simulink model "SAME5x_EXpicGUI_base"  (R2020b)
(part 2 of 3)

      mask TypeOptions FPLLMULT: PLL Multiply by 128 | PLL Multiply by 127 | PLL Multiply by 126 | PLL Multiply by 125 | PLL Multiply by 124 | PLL Multiply by 123 | PLL Multiply by 122 | PLL Multiply by 121 | PLL Multiply by 120 | PLL Multiply by 119 | PLL Multiply by 118 | PLL Multiply by 117 | PLL Multiply by 116 | PLL Multiply by 115 | PLL Multiply by 114 | PLL Multiply by 113 | PLL Multiply by 112 | PLL Multiply by 111 | PLL Multiply by 110 | PLL Multiply by 109 | PLL Multiply by 108 | PLL Multiply by 107 | PLL Multiply by 106 | PLL Multiply by 105 | PLL Multiply by 104 | PLL Multiply by 103 | PLL Multiply by 102 | PLL Multiply by 101 | PLL Multiply by 100 | PLL Multiply by 99 | PLL Multiply by 98 | PLL Multiply by 97 | PLL Multiply by 96 | PLL Multiply by 95 | PLL Multiply by 94 | PLL Multiply by 93 | PLL Multiply by 92 | PLL Multiply by 91 | PLL Multiply by 90 | PLL Multiply by 89 | PLL Multiply by 88 | PLL Multiply by 87 | PLL Multiply by 86 | PLL Multiply by 85 | PLL Multiply by 84 | PLL Multiply by 83 | PLL Multiply by 82 | PLL Multiply by 81 | PLL Multiply by 80 | PLL Multiply by 79 | PLL Multiply by 78 | PLL Multiply by 77 | PLL Multiply by 76 | PLL Multiply by 75 | PLL Multiply by 74 | PLL Multiply by 73 | PLL Multiply by 72 | PLL Multiply by 71 | PLL Multiply by 70 | PLL Multiply by 69 | PLL Multiply by 68 | PLL Multiply by 67 | PLL Multiply by 66 | PLL Multiply by 65 | PLL Multiply by 64 | PLL Multiply by 63 | PLL Multiply by 62 | PLL Multiply by 61 | PLL Multiply by 60 | PLL Multiply by 59 | PLL Multiply by 58 | PLL Multiply by 57 | PLL Multiply by 56 | PLL Multiply by 55 | PLL Multiply by 54 | PLL Multiply by 53 | PLL Multiply by 52 | PLL Multiply by 51 | PLL Multiply by 50 | PLL Multiply by 49 | PLL Multiply by 48 | PLL Multiply by 47 | PLL Multiply by 46 | PLL Multiply by 45 | PLL Multiply by 44 | PLL Multiply by 43 | PLL Multiply by 42 | PLL Multiply by 41 | PLL Multiply by 40 | PLL Multiply by 39 | PLL Multiply by 38 | PLL Multiply by 37 | PLL Multiply by 36 | PLL Multiply by 35 | PLL Multiply by 34 | PLL Multiply by 33 | PLL Multiply by 32 | PLL Multiply by 31 | PLL Multiply by 30 | PLL Multiply by 29 | PLL Multiply by 28 | PLL Multiply by 27 | PLL Multiply by 26 | PLL Multiply by 25 | PLL Multiply by 24 | PLL Multiply by 23 | PLL Multiply by 22 | PLL Multiply by 21 | PLL Multiply by 20 | PLL Multiply by 19 | PLL Multiply by 18 | PLL Multiply by 17 | PLL Multiply by 16 | PLL Multiply by 15 | PLL Multiply by 14 | PLL Multiply by 13 | PLL Multiply by 12 | PLL Multiply by 11 | PLL Multiply by 10 | PLL Multiply by 9 | PLL Multiply by 8 | PLL Multiply by 7 | PLL Multiply by 6 | PLL Multiply by 5 | PLL Multiply by 4 | PLL Multiply by 3 | PLL Multiply by 2 | PLL Multiply by 1
      mask TypeOptions UPLLFSEL: USB PLL input is 24 MHz | USB PLL input is 12 MHz
      mask TypeOptions DMTINTV: Window/Interval value is 127/128 counter value | Window/Interval value is 63/64 counter value | Window/Interval value is 31/32 counter value | Window/Interval value is 15/16 counter value | Window/Interval value is 7/8 counter value | Window/Interval value is 3/4 counter value | Window/Interval value is 1/2 counter value | Window/Interval value is zero
      mask TypeOptions WDTSPGM: WDT stops during Flash programming | WDT runs during Flash programming
      mask TypeOptions FDMTEN: Deadman Timer is enabled | Deadman Timer is disabled
      mask TypeOptions TRCEN: Trace features in the CPU are enabled | Trace features in the CPU are disabled
      mask TypeOptions BOOTISA: Boot code and Exception code is MIPS32 | Boot code and Exception code is microMIPS
      mask TypeOptions FECCCON: ECC and Dynamic ECC are disabled (ECCCON<1:0> bits are writable) | ECC and Dynamic ECC are disabled (ECCCON<1:0> bits are locked) | Dynamic Flash ECC is enabled (ECCCON<1:0> bits are locked) | Flash ECC is enabled (ECCCON<1:0> bits are locked; disables word Flash writes) | ECC and Dynamic ECC are disabled (ECCCON bits are writable) | ECC and Dynamic ECC are disabled (ECCCON bits are locked) | Dynamic Flash ECC is enabled (ECCCON bits are locked) | Flash ECC is enabled (ECCCON bits are locked)
      mask TypeOptions EXTDDRSIZE: Not used
      mask TypeOptions FSLEEP: Flash is powered down when the device is in Sleep mode | Flash power down is controlled by the VREGS bit
      mask TypeOptions DBGPER: Allow CPU access to all permission regions | PG0: Deny PG1: Allow PG2: Allow | PG0: Allow PG1: Deny PG2: Allow | Allow CPU access to Permission Group 2 permission regions | PG0: Allow PG1: Allow PG2: Deny | Allow CPU access to Permission Group 1 permission regions | Allow CPU access to Permission Group 0 permission regions | Deny CPU access to all permission regions
      mask TypeOptions EJTAGBEN: Normal EJTAG functionality | Reduced EJTAG functionality
      mask TypeOptions TSEQ: Not used
      mask TypeOptions CSEQ: Not used
      mask TypeOptions RWDTPS: 1:1048576 | 1:524288 | 1:262144 | 1:131072 | 1:65536 | 1:32768 | 1:16384 | 1:8192 | 1:4096 | 1:2048 | 1:1024 | 1:512 | 1:256 | 1:128 | 1:64 | 1:32 | 1:16 | 1:8 | 1:4 | 1:2 | 1:1 | 1:2147483648 | 1:1073741824 | 1:536870912 | 1:268435456 | 1:134217728 | 1:67108864 | 1:33554432 | 1:16777216 | 1:8388608 | 1:4194304 | 1:2097152
      mask TypeOptions RCLKSEL: Always use LPRC | Use FRC when WINDIS = 0; system clock is not INTOSC/LPRC and device is not in Sleep;otherwise; use INTOSC/LPRC | Use peripheral clk when system clock is not INTOSC/LPRC and device is not in Sleep;otherwise; use INTOSC/LPRC | Always use BFRC/256 | Use FRC when WINDIS = 0 and device is not in Sleep; otherwise; use BFRC/256 | Use peripheral clk when device is not in Sleep; otherwise; use BFRC/256
      mask TypeOptions SWDTPS: 1:1048576 | 1:524288 | 1:262144 | 1:131072 | 1:65536 | 1:32768 | 1:16384 | 1:8192 | 1:4096 | 1:2048 | 1:1024 | 1:512 | 1:256 | 1:128 | 1:64 | 1:32 | 1:16 | 1:8 | 1:4 | 1:2 | 1:1 | 1:2147483648 | 1:1073741824 | 1:536870912 | 1:268435456 | 1:134217728 | 1:67108864 | 1:33554432 | 1:16777216 | 1:8388608 | 1:4194304 | 1:2097152
      mask TypeOptions DMTIVTL: Not used
      mask TypeOptions DMTIVTH: Not used
      mask TypeOptions DMTCNTL: Not used
      mask TypeOptions DMTCNTH: Not used
      mask TypeOptions DMTDIS: Dead Man Timer is Disabled and can be enabled by software | Dead Man Timer is Enabled and cannot be disabled by software
      mask TypeOptions SMBEN: SMBus input threshold is enabled | Standard I2C input threshold operation
      mask TypeOptions SPI2PIN: SPI2 uses I/O remap (PPS) pins | SPI2 uses dedicated I/O pins
      mask TypeOptions CTXT3: Not Assigned | Alternate Register set assigned to IPL level 7 | Alternate Register set assigned to IPL level 6 | Alternate Register set assigned to IPL level 5 | Alternate Register set assigned to IPL level 4 | Alternate Register set assigned to IPL level 3 | Alternate Register set assigned to IPL level 2 | Alternate Register set assigned to IPL level 1
      mask TypeOptions CTXT4: Not Assigned | Alternate Register set assigned to IPL level 7 | Alternate Register set assigned to IPL level 6 | Alternate Register set assigned to IPL level 5 | Alternate Register set assigned to IPL level 4 | Alternate Register set assigned to IPL level 3 | Alternate Register set assigned to IPL level 2 | Alternate Register set assigned to IPL level 1
      mask TypeOptions MBXM0: Mailbox register configured for Master data read (Slave to Master data transfer) | Mailbox register configured for Master data write (Master to Slave data transfer)
      mask TypeOptions MBXM1: Mailbox register configured for Master data read (Slave to Master data transfer) | Mailbox register configured for Master data write (Master to Slave data transfer)
      mask TypeOptions MBXM2: Mailbox register configured for Master data read (Slave to Master data transfer) | Mailbox register configured for Master data write (Master to Slave data transfer)
      mask TypeOptions MBXM3: Mailbox register configured for Master data read (Slave to Master data transfer) | Mailbox register configured for Master data write (Master to Slave data transfer)
      mask TypeOptions MBXM4: Mailbox register configured for Master data read (Slave to Master data transfer) | Mailbox register configured for Master data write (Master to Slave data transfer)
      mask TypeOptions MBXM5: Mailbox register configured for Master data read (Slave to Master data transfer) | Mailbox register configured for Master data write (Master to Slave data transfer)
      mask TypeOptions MBXM6: Mailbox register configured for Master data read (Slave to Master data transfer) | Mailbox register configured for Master data write (Master to Slave data transfer)
      mask TypeOptions MBXM7: Mailbox register configured for Master data read (Slave to Master data transfer) | Mailbox register configured for Master data write (Master to Slave data transfer)
      mask TypeOptions MBXM8: Mailbox register configured for Master data read (Slave to Master data transfer) | Mailbox register configured for Master data write (Master to Slave data transfer)
      mask TypeOptions MBXM9: Mailbox register configured for Master data read (Slave to Master data transfer) | Mailbox register configured for Master data write (Master to Slave data transfer)
      mask TypeOptions MBXM10: Mailbox register configured for Master data read (Slave to Master data transfer) | Mailbox register configured for Master data write (Master to Slave data transfer)
      mask TypeOptions MBXM11: Mailbox register configured for Master data read (Slave to Master data transfer) | Mailbox register configured for Master data write (Master to Slave data transfer)
      mask TypeOptions MBXM12: Mailbox register configured for Master data read (Slave to Master data transfer) | Mailbox register configured for Master data write (Master to Slave data transfer)
      mask TypeOptions MBXM13: Mailbox register configured for Master data read (Slave to Master data transfer) | Mailbox register configured for Master data write (Master to Slave data transfer)
      mask TypeOptions MBXM14: Mailbox register configured for Master data read (Slave to Master data transfer) | Mailbox register configured for Master data write (Master to Slave data transfer)
      mask TypeOptions MBXM15: Mailbox register configured for Master data read (Slave to Master data transfer) | Mailbox register configured for Master data write (Master to Slave data transfer)
      mask TypeOptions MBXHSA: MSIxMBXD15 assigned to mailbox handshake protocol block A | MSIxMBXD14 assigned to mailbox handshake protocol block A | MSIxMBXD13 assigned to mailbox handshake protocol block A | MSIxMBXD12 assigned to mailbox handshake protocol block A | MSIxMBXD11 assigned to mailbox handshake protocol block A | MSIxMBXD10 assigned to mailbox handshake protocol block A | MSIxMBXD9 assigned to mailbox handshake protocol block A | MSIxMBXD8 assigned to mailbox handshake protocol block A | MSIxMBXD7 assigned to mailbox handshake protocol block A | MSIxMBXD6 assigned to mailbox handshake protocol block A | MSIxMBXD5 assigned to mailbox handshake protocol block A | MSIxMBXD4 assigned to mailbox handshake protocol block A | MSIxMBXD3 assigned to mailbox handshake protocol block A | MSIxMBXD2 assigned to mailbox handshake protocol block A | MSIxMBXD1 assigned to mailbox handshake protocol block A | MSIxMBXD0 assigned to mailbox handshake protocol block A
      mask TypeOptions MBXHSB: MSIxMBXD15 assigned to mailbox handshake protocol block B | MSIxMBXD14 assigned to mailbox handshake protocol block B | MSIxMBXD13 assigned to mailbox handshake protocol block B | MSIxMBXD12 assigned to mailbox handshake protocol block B | MSIxMBXD11 assigned to mailbox handshake protocol block B | MSIxMBXD10 assigned to mailbox handshake protocol block B | MSIxMBXD9 assigned to mailbox handshake protocol block B | MSIxMBXD8 assigned to mailbox handshake protocol block B | MSIxMBXD7 assigned to mailbox handshake protocol block B | MSIxMBXD6 assigned to mailbox handshake protocol block B | MSIxMBXD5 assigned to mailbox handshake protocol block B | MSIxMBXD4 assigned to mailbox handshake protocol block B | MSIxMBXD3 assigned to mailbox handshake protocol block B | MSIxMBXD2 assigned to mailbox handshake protocol block B | MSIxMBXD1 assigned to mailbox handshake protocol block B | MSIxMBXD0 assigned to mailbox handshake protocol block B
      mask TypeOptions MBXHSC: MSIxMBXD15 assigned to mailbox handshake protocol block C | MSIxMBXD14 assigned to mailbox handshake protocol block C | MSIxMBXD13 assigned to mailbox handshake protocol block C | MSIxMBXD12 assigned to mailbox handshake protocol block C | MSIxMBXD11 assigned to mailbox handshake protocol block C | MSIxMBXD10 assigned to mailbox handshake protocol block C | MSIxMBXD9 assigned to mailbox handshake protocol block C | MSIxMBXD8 assigned to mailbox handshake protocol block C | MSIxMBXD7 assigned to mailbox handshake protocol block C | MSIxMBXD6 assigned to mailbox handshake protocol block C | MSIxMBXD5 assigned to mailbox handshake protocol block C | MSIxMBXD4 assigned to mailbox handshake protocol block C | MSIxMBXD3 assigned to mailbox handshake protocol block C | MSIxMBXD2 assigned to mailbox handshake protocol block C | MSIxMBXD1 assigned to mailbox handshake protocol block C | MSIxMBXD0 assigned to mailbox handshake protocol block C
      mask TypeOptions MBXHSD: MSIxMBXD15 assigned to mailbox handshake protocol block D | MSIxMBXD14 assigned to mailbox handshake protocol block D | MSIxMBXD13 assigned to mailbox handshake protocol block D | MSIxMBXD12 assigned to mailbox handshake protocol block D | MSIxMBXD11 assigned to mailbox handshake protocol block D | MSIxMBXD10 assigned to mailbox handshake protocol block D | MSIxMBXD9 assigned to mailbox handshake protocol block D | MSIxMBXD8 assigned to mailbox handshake protocol block D | MSIxMBXD7 assigned to mailbox handshake protocol block D | MSIxMBXD6 assigned to mailbox handshake protocol block D | MSIxMBXD5 assigned to mailbox handshake protocol block D | MSIxMBXD4 assigned to mailbox handshake protocol block D | MSIxMBXD3 assigned to mailbox handshake protocol block D | MSIxMBXD2 assigned to mailbox handshake protocol block D | MSIxMBXD1 assigned to mailbox handshake protocol block D | MSIxMBXD0 assigned to mailbox handshake protocol block D
      mask TypeOptions MBXHSE: MSIxMBXD15 assigned to mailbox handshake protocol block E | MSIxMBXD14 assigned to mailbox handshake protocol block E | MSIxMBXD13 assigned to mailbox handshake protocol block E | MSIxMBXD12 assigned to mailbox handshake protocol block E | MSIxMBXD11 assigned to mailbox handshake protocol block E | MSIxMBXD10 assigned to mailbox handshake protocol block E | MSIxMBXD9 assigned to mailbox handshake protocol block E | MSIxMBXD8 assigned to mailbox handshake protocol block E | MSIxMBXD7 assigned to mailbox handshake protocol block E | MSIxMBXD6 assigned to mailbox handshake protocol block E | MSIxMBXD5 assigned to mailbox handshake protocol block E | MSIxMBXD4 assigned to mailbox handshake protocol block E | MSIxMBXD3 assigned to mailbox handshake protocol block E | MSIxMBXD2 assigned to mailbox handshake protocol block E | MSIxMBXD1 assigned to mailbox handshake protocol block E | MSIxMBXD0 assigned to mailbox handshake protocol block E
      mask TypeOptions MBXHSF: MSIxMBXD15 assigned to mailbox handshake protocol block F | MSIxMBXD14 assigned to mailbox handshake protocol block F | MSIxMBXD13 assigned to mailbox handshake protocol block F | MSIxMBXD12 assigned to mailbox handshake protocol block F | MSIxMBXD11 assigned to mailbox handshake protocol block F | MSIxMBXD10 assigned to mailbox handshake protocol block F | MSIxMBXD9 assigned to mailbox handshake protocol block F | MSIxMBXD8 assigned to mailbox handshake protocol block F | MSIxMBXD7 assigned to mailbox handshake protocol block F | MSIxMBXD6 assigned to mailbox handshake protocol block F | MSIxMBXD5 assigned to mailbox handshake protocol block F | MSIxMBXD4 assigned to mailbox handshake protocol block F | MSIxMBXD3 assigned to mailbox handshake protocol block F | MSIxMBXD2 assigned to mailbox handshake protocol block F | MSIxMBXD1 assigned to mailbox handshake protocol block F | MSIxMBXD0 assigned to mailbox handshake protocol block F
      mask TypeOptions MBXHSG: MSIxMBXD15 assigned to mailbox handshake protocol block G | MSIxMBXD14 assigned to mailbox handshake protocol block G | MSIxMBXD13 assigned to mailbox handshake protocol block G | MSIxMBXD12 assigned to mailbox handshake protocol block G | MSIxMBXD11 assigned to mailbox handshake protocol block G | MSIxMBXD10 assigned to mailbox handshake protocol block G | MSIxMBXD9 assigned to mailbox handshake protocol block G | MSIxMBXD8 assigned to mailbox handshake protocol block G | MSIxMBXD7 assigned to mailbox handshake protocol block G | MSIxMBXD6 assigned to mailbox handshake protocol block G | MSIxMBXD5 assigned to mailbox handshake protocol block G | MSIxMBXD4 assigned to mailbox handshake protocol block G | MSIxMBXD3 assigned to mailbox handshake protocol block G | MSIxMBXD2 assigned to mailbox handshake protocol block G | MSIxMBXD1 assigned to mailbox handshake protocol block G | MSIxMBXD0 assigned to mailbox handshake protocol block G
      mask TypeOptions MBXHSH: MSIxMBXD15 assigned to mailbox handshake protocol block H | MSIxMBXD14 assigned to mailbox handshake protocol block H | MSIxMBXD13 assigned to mailbox handshake protocol block H | MSIxMBXD12 assigned to mailbox handshake protocol block H | MSIxMBXD11 assigned to mailbox handshake protocol block H | MSIxMBXD10 assigned to mailbox handshake protocol block H | MSIxMBXD9 assigned to mailbox handshake protocol block H | MSIxMBXD8 assigned to mailbox handshake protocol block H | MSIxMBXD7 assigned to mailbox handshake protocol block H | MSIxMBXD6 assigned to mailbox handshake protocol block H | MSIxMBXD5 assigned to mailbox handshake protocol block H | MSIxMBXD4 assigned to mailbox handshake protocol block H | MSIxMBXD3 assigned to mailbox handshake protocol block H | MSIxMBXD2 assigned to mailbox handshake protocol block H | MSIxMBXD1 assigned to mailbox handshake protocol block H | MSIxMBXD0 assigned to mailbox handshake protocol block H
      mask TypeOptions HSAEN: Mailbox data flow control handshake protocol block disabled. | Mailbox data flow control handshake protocol block enabled
      mask TypeOptions HSBEN: Mailbox data flow control handshake protocol block disabled. | Mailbox data flow control handshake protocol block enabled
      mask TypeOptions HSCEN: Mailbox data flow control handshake protocol block disabled. | Mailbox data flow control handshake protocol block enabled
      mask TypeOptions HSDEN: Mailbox data flow control handshake protocol block disabled. | Mailbox data flow control handshake protocol block enabled
      mask TypeOptions HSEEN: Mailbox data flow control handshake protocol block disabled. | Mailbox data flow control handshake protocol block enabled
      mask TypeOptions HSFEN: Mailbox data flow control handshake protocol block disabled. | Mailbox data flow control handshake protocol block enabled
      mask TypeOptions HSGEN: Mailbox data flow control handshake protocol block disabled. | Mailbox data flow control handshake protocol block enabled
      mask TypeOptions HSHEN: Mailbox data flow control handshake protocol block disabled. | Mailbox data flow control handshake protocol block enabled
      mask TypeOptions CPRA0: Master core owns pin. | Slave 1 core owns pin.
      mask TypeOptions CPRA1: Master core owns pin. | Slave 1 core owns pin.
      mask TypeOptions CPRA2: Master core owns pin. | Slave 1 core owns pin.
      mask TypeOptions CPRA3: Master core owns pin. | Slave 1 core owns pin.
      mask TypeOptions CPRA4: Master core owns pin. | Slave 1 core owns pin.
      mask TypeOptions CPRB0: Master core owns pin. | Slave 1 core owns pin.
      mask TypeOptions CPRB1: Master core owns pin. | Slave 1 core owns pin.
      mask TypeOptions CPRB2: Master core owns pin. | Slave 1 core owns pin.
      mask TypeOptions CPRB3: Master core owns pin. | Slave 1 core owns pin.
      mask TypeOptions CPRB4: Master core owns pin. | Slave 1 core owns pin.
      mask TypeOptions CPRB5: Master core owns pin. | Slave 1 core owns pin.
      mask TypeOptions CPRB6: Master core owns pin. | Slave 1 core owns pin.
      mask TypeOptions CPRB7: Master core owns pin. | Slave 1 core owns pin.
      mask TypeOptions CPRB8: Master core owns pin. | Slave 1 core owns pin.
      mask TypeOptions CPRB9: Master core owns pin. | Slave 1 core owns pin.
      mask TypeOptions CPRB10: Master core owns pin. | Slave 1 core owns pin.
      mask TypeOptions CPRB11: Master core owns pin. | Slave 1 core owns pin.
      mask TypeOptions CPRB12: Master core owns pin. | Slave 1 core owns pin.
      mask TypeOptions CPRB13: Master core owns pin. | Slave 1 core owns pin.
      mask TypeOptions CPRB14: Master core owns pin. | Slave 1 core owns pin.
      mask TypeOptions CPRB15: Master core owns pin. | Slave 1 core owns pin.
      mask TypeOptions CPRC0: Master core owns pin. | Slave 1 core owns pin.
      mask TypeOptions CPRC1: Master core owns pin. | Slave 1 core owns pin.
      mask TypeOptions CPRC2: Master core owns pin. | Slave 1 core owns pin.
      mask TypeOptions CPRC3: Master core owns pin. | Slave 1 core owns pin.
      mask TypeOptions CPRC4: Master core owns pin. | Slave 1 core owns pin.
      mask TypeOptions CPRC5: Master core owns pin. | Slave 1 core owns pin.
      mask TypeOptions CPRC6: Master core owns pin. | Slave 1 core owns pin.
      mask TypeOptions CPRC7: Master core owns pin. | Slave 1 core owns pin.
      mask TypeOptions CPRC8: Master core owns pin. | Slave 1 core owns pin.
      mask TypeOptions CPRC9: Master core owns pin. | Slave 1 core owns pin.
      mask TypeOptions CPRC10: Master core owns pin. | Slave 1 core owns pin.
      mask TypeOptions CPRC11: Master core owns pin. | Slave 1 core owns pin.
      mask TypeOptions CPRC12: Master core owns pin. | Slave 1 core owns pin.
      mask TypeOptions CPRC13: Master core owns pin. | Slave 1 core owns pin.
      mask TypeOptions CPRC14: Master core owns pin. | Slave 1 core owns pin.
      mask TypeOptions CPRC15: Master core owns pin. | Slave 1 core owns pin.
      mask TypeOptions CPRD0: Master core owns pin. | Slave 1 core owns pin.
      mask TypeOptions CPRD1: Master core owns pin. | Slave 1 core owns pin.
      mask TypeOptions CPRD2: Master core owns pin. | Slave 1 core owns pin.
      mask TypeOptions CPRD3: Master core owns pin. | Slave 1 core owns pin.
      mask TypeOptions CPRD4: Master core owns pin. | Slave 1 core owns pin.
      mask TypeOptions CPRD5: Master core owns pin. | Slave 1 core owns pin.
      mask TypeOptions CPRD6: Master core owns pin. | Slave 1 core owns pin.
      mask TypeOptions CPRD7: Master core owns pin. | Slave 1 core owns pin.
      mask TypeOptions CPRD8: Master core owns pin. | Slave 1 core owns pin.
      mask TypeOptions CPRD9: Master core owns pin. | Slave 1 core owns pin.
      mask TypeOptions CPRD10: Master core owns pin. | Slave 1 core owns pin.
      mask TypeOptions CPRD11: Master core owns pin. | Slave 1 core owns pin.
      mask TypeOptions CPRD12: Master core owns pin. | Slave 1 core owns pin.
      mask TypeOptions CPRD13: Master core owns pin. | Slave 1 core owns pin.
      mask TypeOptions CPRD14: Master core owns pin. | Slave 1 core owns pin.
      mask TypeOptions CPRD15: Master core owns pin. | Slave 1 core owns pin.
      mask TypeOptions CPRE0: Master core owns pin. | Slave 1 core owns pin.
      mask TypeOptions CPRE1: Master core owns pin. | Slave 1 core owns pin.
      mask TypeOptions CPRE2: Master core owns pin. | Slave 1 core owns pin.
      mask TypeOptions CPRE3: Master core owns pin. | Slave 1 core owns pin.
      mask TypeOptions CPRE4: Master core owns pin. | Slave 1 core owns pin.
      mask TypeOptions CPRE5: Master core owns pin. | Slave 1 core owns pin.
      mask TypeOptions CPRE6: Master core owns pin. | Slave 1 core owns pin.
      mask TypeOptions CPRE7: Master core owns pin. | Slave 1 core owns pin.
      mask TypeOptions CPRE8: Master core owns pin. | Slave 1 core owns pin.
      mask TypeOptions CPRE9: Master core owns pin. | Slave 1 core owns pin.
      mask TypeOptions CPRE10: Master core owns pin. | Slave 1 core owns pin.
      mask TypeOptions CPRE11: Master core owns pin. | Slave 1 core owns pin.
      mask TypeOptions CPRE12: Master core owns pin. | Slave 1 core owns pin.
      mask TypeOptions CPRE13: Master core owns pin. | Slave 1 core owns pin.
      mask TypeOptions CPRE14: Master core owns pin. | Slave 1 core owns pin.
      mask TypeOptions CPRE15: Master core owns pin. | Slave 1 core owns pin.
      mask TypeOptions S1FNOSC: Internal Fast RC (FRC) Oscillator with postscaler | Back up Fast RC (BFRC) Oscillator | Low-Power RC Oscillator (LPRC) | Primary Oscillator with PLL module (XT + PLL; HS + PLL; EC + PLL) | Primary Oscillator (XT; HS; EC) | Fast RC Oscillator with divide-by-N with PLL module (FRCPLL)  | Internal Fast RC (FRC)
      mask TypeOptions S1IESO: Start up with FRC; then switch | Disable
      mask TypeOptions S1OSCIOFNC: OSC2 is clock output | general purpose digital I/O pin
      mask TypeOptions S1FCKSM: Both Clock switching and Fail-safe Clock Monitor are disabled | Clock switching is enabled;Fail-safe Clock Monitor is disabled | Both Clock switching and Fail-safe Clock Monitor are enabled
      mask TypeOptions S1PLLKEN: S1PLLKEN_ON | S1PLLKEN_OFF
      mask TypeOptions S1RWDTPS: 1:1048576 | 1:524288 | 1:262144 | 1:131072 | 1:65536 | 1:32768 | 1:16384 | 1:8192 | 1:4096 | 1:2048 | 1:1024 | 1:512 | 1:256 | 1:128 | 1:64 | 1:32 | 1:16 | 1:8 | 1:4 | 1:2 | 1:1
      mask TypeOptions S1RCLKSEL: Always use LPRC | Use FRC when WINDIS = 0; system clock is not INTOSC/LPRC and device is not in Sleep; otherwise; use INTOSC/LPRC | Use peripheral clk when system clock is not INTOSC/LPRC and device is not in Sleep;otherwise; use INTOSC/LPRC
      mask TypeOptions S1WINDIS: Watchdog Timer operates in Non-Window mode | Watchdog Timer operates in Window mode
      mask TypeOptions S1WDTWIN: WDT Window is 25% of WDT period | WDT Window is 37.5% of WDT period | WDT Window is 50% of WDT period | WDT Windo is 75% of WDT period
      mask TypeOptions S1SWDTPS: 1:1048576 | 1:524288 | 1:262144 | 1:131072 | 1:65536 | 1:32768 | 1:16384 | 1:8192 | 1:4096 | 1:2048 | 1:1024 | 1:512 | 1:256 | 1:128 | 1:64 | 1:32 | 1:16 | 1:8 | 1:4 | 1:2 | 1:1
      mask TypeOptions S1FWDTEN: Enable | Disable
      mask TypeOptions S1ICS: Communicate on PGC1 and PGD1 | Communicate on PGC2 and PGD2 | Communicate on PGC3 and PGD3
      mask TypeOptions S1DEBUG: Not used
      mask TypeOptions S1ISOLAT: The slave can operate (in debug mode) even if the SLVEN bit in the MSI is zero. | The slave can only operate if the SLVEN bit in the MSI is set.
      mask TypeOptions S1NOBTSWP: BOOTSWP instruction is disabled | BOOTSWP instruction is enabled
      mask TypeOptions S1ALTI2C1: I2C1 mapped to SDA1/SCL1 pins | I2C1 mapped to ASDA1/ASCL1 pins
      mask TypeOptions S1SPI1PIN: Slave SPI1 uses I/O remap (PPS) pins | Slave SPI1 uses dedicated I/O pins
      mask TypeOptions S1SSRE: Slave generated resets will reset the Slave Enable Bit in the MSI module | Slave generated resets will not reset the Slave Enable Bit in the MSI module
      mask TypeOptions S1MSRE: The master software oriented RESET events (RESET Op-Code; Watchdog timeout; TRAP reset; illegalInstruction) will also cause the slave subsystem to reset. | The master software oriented RESET events (RESET Op-Code; Watchdog timeout; TRAP reset; illegalInstruction) will not cause the slave subsystem to reset.
      mask TypeOptions S1CTXT1: Not Assigned | Alternate Register set assigned to IPL level 7 | Alternate Register set assigned to IPL level 6 | Alternate Register set assigned to IPL level 5 | Alternate Register set assigned to IPL level 4 | Alternate Register set assigned to IPL level 3 | Alternate Register set assigned to IPL level 2 | Alternate Register set assigned to IPL level 1
      mask TypeOptions S1CTXT2: Not Assigned | Alternate Register set assigned to IPL level 7 | Alternate Register set assigned to IPL level 6 | Alternate Register set assigned to IPL level 5 | Alternate Register set assigned to IPL level 4 | Alternate Register set assigned to IPL level 3 | Alternate Register set assigned to IPL level 2 | Alternate Register set assigned to IPL level 1
      mask TypeOptions S1CTXT3: Not Assigned | Alternate Register set assigned to IPL level 7 | Alternate Register set assigned to IPL level 6 | Alternate Register set assigned to IPL level 5 | Alternate Register set assigned to IPL level 4 | Alternate Register set assigned to IPL level 3 | Alternate Register set assigned to IPL level 2 | Alternate Register set assigned to IPL level 1
      mask TypeOptions S1CTXT4: Not Assigned | Alternate Register set assigned to IPL level 7 | Alternate Register set assigned to IPL level 6 | Alternate Register set assigned to IPL level 5 | Alternate Register set assigned to IPL level 4 | Alternate Register set assigned to IPL level 3 | Alternate Register set assigned to IPL level 2 | Alternate Register set assigned to IPL level 1
      mask TypeOptions BORLVL: Not used
      mask TypeOptions BSSO: Not used
      mask TypeOptions MCA: Not used
      mask TypeOptions MAXTEMP: Not used
      mask TypeOptions CFGAN14: Not used
      mask TypeOptions CFGAN15: Not used
      mask TypeOptions S1IOL1WAY: Not used
      mask TypeOptions S1BSSO: Not used
      mask TypeOptions S1BACKBUG: Not used
      mask TypeOptions BISTDIS: mBIST on reset feature disabled | mBIST on reset feature enabled
      mask TypeOptions NOBTSWP: BOOTSWP instruction is disabled | BOOTSWP instruction is enabled
      mask TypeOptions S1BISTDIS: Slave BIST on reset feature disabled | Slave BIST on reset feature enabled
      mask TypeOptions S1DMTIVTL: Not used
      mask TypeOptions S1DMTIVTH: Not used
      mask TypeOptions S1DMTCNTL: Not used
      mask TypeOptions S1DMTCNTH: Not used
      mask TypeOptions S1DMTDIS: Slave Dead Man Timer is Disabled and can be enabled by software | Slave Dead Man Timer is Enabled and cannot be disabled by software
      mask TypeOptions BSEQ: Not used
      mask TypeOptions IBSEQ: Not used
      mask TypeOptions SMB3EN: SMBus 3.0 input levels | Normal  SMBus input levels
      mask TypeOptions FUSBIDIO2: USBID pin is controlled by the USB2 module | USBID pin is controlled by the port function
      mask TypeOptions FVBUSIO2: VBUSON pin is controlled by the USB2 module | VBUSON pin is controlled by the port function
      mask TypeOptions FUSBIDIO1: USBID pin is controlled by the USB1 module | USBID pin is controlled by the port function
      mask TypeOptions FVBUSIO1: VBUSON pin is controlled by the USB1 module | VBUSON pin is controlled by the port function
      mask TypeOptions VBATBOREN: Enable ZPBOR during VBAT Mode | Disable ZPBOR during VBAT Mode
      mask TypeOptions FDSEN: Enable DSEN bit in DSCON | Disable DSEN bit in DSCON
      mask TypeOptions BORSEL: BOR trip voltage 2.1v (Non-OPAMP deviced operation) | BOR trip voltage 2.8v (OPAMP deviced operation)
      mask TypeOptions POSCFGAIN: Gain is G3 | Gain is G2 | Gain is G1 | Gain is G0
      mask TypeOptions POSCAGCDLY: Settling time = 25ms x AGCRNG | Settling time = 6.25ms x AGCRNG | Settling time = 400ms x AGCRNG | Settling time = 100ms x AGCRNG
      mask TypeOptions POSCAGCRNG: Range 1x | Range 5x
      mask TypeOptions POSCAGC: Automatic Gain Control for Oscillator | Manual Gain Control of Oscillator
      mask TypeOptions FDBGWP: Not used
      mask DialogControl ParameterTabVar0 Prompt: General
      mask DialogControl ParameterTabVar01 Prompt: Oscillator
      mask DialogControl ParameterTabVar012 Prompt: Memory
      mask DialogControl ParameterTabVar0123 Prompt: Debug
      mask DialogControl ParameterTabVar01234 Prompt: DualCore
      mask Display: MCHP_DrawLogo;fprintf('MCHP_MASTER\\nSAME54P20A - TQFP128\\n100MHZ');
  Model : Subsystem
  Model Info : simulink/Model-Wide Utilities/Model Info  Frame=on  DisplayStringWithTags=|  HorizontalTextAlignment=Center  LeftAlignmentValue=0.5
      | %<ModelName> v%<ModelVersion> - %<Creator>
      | 
      | %<Description>
      | 
      | Last modified on: %<LastModificationDate>
  "Modes Serial Terminal " : Subsystem
  OR : Logic  Operator=OR  IconShape=distinctive  AllPortsSameDT=off  OutDataTypeStr=boolean
  Port Info : S-Function  FunctionName=MCHP_EmptySFunction  SFunctionDeploymentMode=off  EnableBusSupport=off  mask{MCHP_MASTERLINK=SAME5x_EXpicGUI/Microchip Master}
      mask init:
      | MCHP_PortInfo_Callback(gcbh,'INITIALISATION');
      settings: CopyFcn=MCHP_PortInfo_Callback(gcb,'COPY');  OpenFcn=MCHP_PortInfo_Callback(gcb,'OPEN');
      mask Display: MCHP_DrawLogo;text(.05,20,'[Pin]  Port   -  Desc\n [48]   PD9  -  DIN -  ( Digital In )\n [60]   PA12 -  SERCOM2_PAD0 -  ( UART2 Tx )\n [61]   PA13 -  SERCOM2_PAD1 -  ( UART2 Rx )\n[102]   PB26 -  DOU -  ( Digital Out )','verticalalignment','Top','horizontalalignment','left');text(.95,0.05,'(4 pins)','verticalalignment','Bottom','horizontalalignment','right');
  Rate Transition : RateTransition
  Reference : Subsystem
  UART Configuration1 : MCHP_Blockset/BUS UART/UART Configuration  UART_REF=SERCOM USART 2  BAUD_Choice=Dynamic Options  BAUD_Choice_TXT="921600         [-0.00%]"  BAUD_Choice_IR=Dynamic Options  BAUD_Choice_IR_TXT=[]  BAUD_Custom=115200  INT_PRIORITY=0  ALT_IO=on  PIN_RX=Dynamic Options  PIN_RX_TXT=PA13 / Pin[61] / pad1  PIN_TX=Dynamic Options  PIN_TX_TXT=PA12 / Pin[60] / pad0  MCHP_PORT={UART2 Rx}{SERCOM2_PAD1}3:0:P13;{UART2 Tx}{SERCOM2_PAD0}3:1:P12;  MCHP_MASTERLINK=SAME5x_EXpicGUI_base/Microchip Master  MCHP_COM_ExtPil=off  TX_IMPLEMENTATION=Circular Buffer  TX_IMPLEMENTATION_default=Circular Buffer  TX_INT_PRIORITY=5  TX_INT_WHEN=is empty  TX_INT_WHEN_default=is empty & last char is sent  TX_CIRCULAR_SIZE=128  TX_DMA_CHANNEL=0  TX_DMA_SIZE=[]  TX_TASK_PROTECTION=Delay tasks (default)  TX_INTERRUPT_PROTECTION=Do not send on conflict (default)  TX_INTERRUPT_PROTECTION_default=Do not send on conflict (default)  RX_IMPLEMENTATION=Circular Buffer  RX_IMPLEMENTATION_default=Circular Buffer  RX_INT_PRIORITY=5  RX_INT_WHEN=receive 1 character  RX_CIRCULAR_SIZE=128  RX_DMA_CHANNEL=0  RX_DMA_SIZE=0  DuplexMode=Full duplex (default)  PIN_RX_Inv=off  PIN_TX_Inv=off  PIN_RXTX_Inv=off  ParityBit=No parity (default)  StopBit=1 stop bit (default)  IRDA=off  FlowControl=None  PIN_CTS=Dynamic Options  PIN_CTS_TXT=PA10 / Pin[35] / pad2  PIN_RTS=Dynamic Options  PIN_RTS_TXT=PA11 / Pin[36] / pad3  InitSequence_chkbox=off  BAUD_Choice_InitSeq=Dynamic Options  BAUD_Choice_InitSeq_TXT="110         [+13.30%]"  BAUD_Choice_IR_InitSeq=Dynamic Options  BAUD_Choice_IR_InitSeq_TXT=0  BAUD_Custom_InitSeq=0  InitSequence='Hello World'
      settings: SourceProductName=MPLAB Device Blocks for Simulink
  picgui Graphical interface : MCHP_Blockset/BUS UART/picgui Graphical interface  Nothing=0
      settings: SourceProductName=MPLAB Device Blocks for Simulink
  tag scope: start=global
  wires:
  Counter Limited/1 -> Data Type Conversion/1  "U2 CH1"
  Data Type Conversion/1 -> DBG_LED2/1
  [u] -> DataVisu/2(u)
  [x] -> DataVisu/3(x)
  Model/1(x) -> [x]
  "Modes Serial Terminal "/1(modes) -> [mode]  "U2 CH1"
  [mode] -> Reference/1(mode)
  [mode] -> DataVisu/1(mode)
  BTN_S2/1 -> EnableLog/1(BTN)
  EnableLog/1(EnableLog) -> OR/2
  [start] -> Reference/2(start)
  [start] -> DataVisu/Enable
  Reference/1(ref) -> [u], Model/1(u)
  OR/1 -> [start]
  [mode] -> Rate Transition/1
  Compare To Constant/1 -> OR/1
  Rate Transition/1 -> Compare To Constant/1
